simulink model "Induction_motor_Speed_Control_PI"  (R2023a)
settings: Solver=ode23t  StartTime=0.0  StopTime=3  RelTol=1e-3  EnableMultiTasking=on
InitFcn:
  | f=50;
  | fs=2000;
  | %jj=readfis('jayashree1');
libraries: spsAsynchronousMachineSIUnitsLib x1, spsDCVoltageSourceLib x1, simulink x1, powerlib_extras x1, spsThreePhaseVIMeasurementLib x1, spsUniversalBridgeLib x1, sps_lib x1
settings Model: Creator=admin  LastModifiedBy=ravikrishna_g3
settings SolverCC: ZeroCrossControl=DisableAll  AlgebraicLoopSolver=TrustRegion
settings DataIOCC: LimitDataPoints=on  SaveFormat=Array  SignalLoggingSaveFormat=ModelDataLogs  ReturnWorkspaceOutputs=off
settings OptimizationCC: ExpressionDepthLimit=2147483647  LifeSpan=inf
settings DebuggingCC: UnderspecifiedInitializationDetection=Classic  MergeDetectMultiDrivingBlocksExec=none  SolverPrmCheckMsg=warning  FcnCallInpInsideContextMsg=warning  UnconnectedInputMsg=warning  UnconnectedOutputMsg=warning  UnconnectedLineMsg=warning  StateNameClashWarn=warning  SFUnexpectedBacktrackingDiag=warning  SFNoUnconditionalDefaultTransitionDiag=warning  SFExecutionAtInitializationDiag=none  ArithmeticOperatorsInVariantConditions=warning
settings HardwareCC: ProdBitPerPointer=32  ProdBitPerSizeT=32  ProdBitPerPtrDiffT=32  ProdLargestAtomicFloat=None  ProdIntDivRoundTo=Undefined  ProdEndianess=Unspecified  ProdWordSize=32  ProdHWDeviceType=32-bit Generic
settings ModelReferenceCC: PropagateSignalLabelsOutOfModel=off
settings SFSimCC: SimUseLocalCustomCode=off  CustomCodeUndefinedFunction=UseInterfaceOnly
settings RTWCC: RTWUseLocalCustomCode=off
settings CodeAppCC: StateflowObjectComments=on
settings GRTTargetCC: TargetLangStandard=C89/C90 (ANSI)  CombineOutputUpdateFcns=off  GRTInterface=on
settings ConfigComp: CovMetricSettings=dw  CovSaveCumulativeToWorkspaceVar=on  CovSaveSingleToWorkspaceVar=on  CovExternalEMLEnable=off

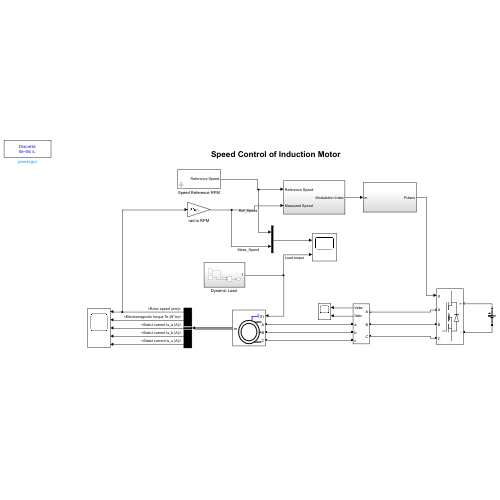
[thumbnail: Simulink's stored preview of the top-level diagram]
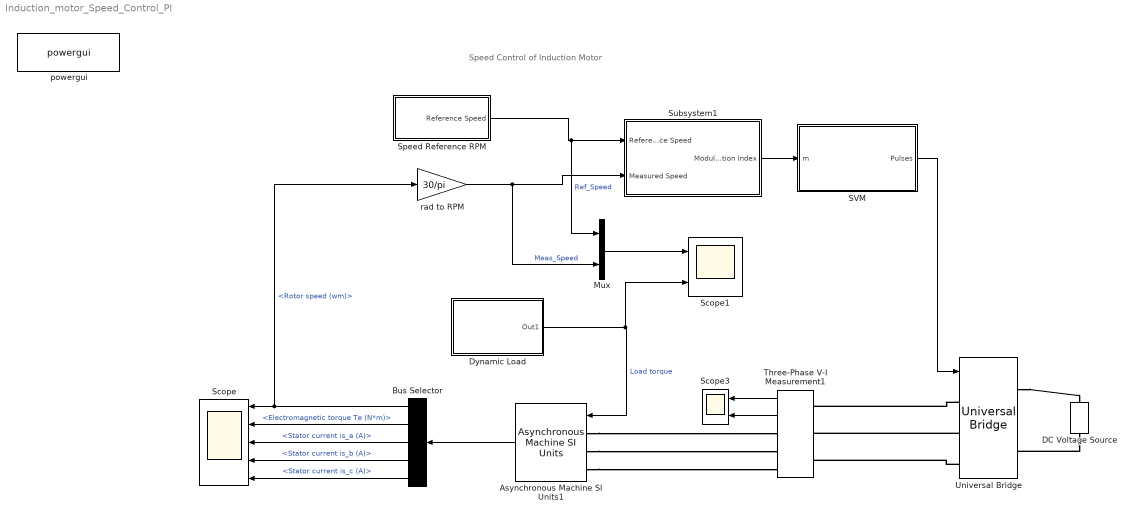
== system Induction_motor_Speed_Control_PI ==
  note: Speed Control of Induction Motor
  Asynchronous Machine SI Units1 : spsAsynchronousMachineSIUnitsLib/Asynchronous Machine SI Units  RotorType=Squirrel-cage  PresetModel="16:  10 HP (7.5KW)  400 V 50Hz 1440 RPM"  MechanicalLoad=Torque Tm  ShowDetailedParameters=on  ReferenceFrame=Rotor  Units=SI  MeasurementBus=off  NominalParameters=[7500 400 50]  VoltageRatio=1  Stator=[0.7384 0.003045]  Rotor=[0.7402 0.003045]  Cage1=[ 0.022 0.226/377]  Cage2=[ 0.022 0.226/377]  Lm=0.1241  Mechanical=[0.0343 0.000503 2]  PolePairs=2  InitialConditions=[1 0 0 0 0 0 0 0]  SimulateSaturation=off  Saturation=[14.03593122, 27.81365428, 53.79336849, 72.68890987, 97.98006896, 148.6815601, 215.7428561, 302.9841135, 428.7778367 ; 230, 322, 414, 460, 506, 552, 598, 644, 690]  LoadFlowParameters=1492000  TsPowergui=0  TsBlock=-1  IterativeModel=Forward Euler  IterativeDiscreteModel=Trapezoidal non iterative  Pmec=0
      settings: AttributesFormatString=\n
  Bus Selector : BusSelector  OutputSignals=Mechanical.Rotor speed (wm),Mechanical.Electromagnetic torque Te (N*m),Stator measurements.Stator current is_a (A),Stator measurements.Stator current is_b (A),Stator measurements.Stator current is_c (A)
  DC Voltage Source : spsDCVoltageSourceLib/DC Voltage Source  Amplitude=400  Measurements=None
  "Dynamic Load " : Subsystem
  Mux : Mux  Inputs=2
  SVM : Subsystem
  Scope : Scope  NumInputPorts=5
  Scope1 : Scope  NumInputPorts=2
  Scope3 : Scope  NumInputPorts=2
  Speed Reference RPM : Subsystem
      mask DialogControl DescTextVar Prompt: Speed
  Subsystem1 : Subsystem
  Three-Phase V-I Measurement1 : spsThreePhaseVIMeasurementLib/Three-Phase V-I Measurement  VoltageMeasurement=phase-to-phase  SetLabelV=off  LabelV=Vabc  Vpu=off  VpuLL=off  CurrentMeasurement=yes  SetLabelI=off  LabelI=Iabc  Ipu=off  Pbase=100e6  Vbase=500e3  OutputType=Complex  PhasorSimulation=off  PSBequivalent=0
  Universal Bridge : spsUniversalBridgeLib/Universal Bridge  Arms=3  SnubberResistance=500  SnubberCapacitance=1e-6  Device=MOSFET / Diodes  Ron=1e-6  Lon=0  ForwardVoltages="[  0  0  ]"  ForwardVoltage=0  GTOparameters=[ 10e-6 , 20e-6 ]  IGBTparameters=[ 1e-6 , 2e-6 ]  Measurements=None  Measurements_2=None  converterType=Rectifier
  powergui : sps_lib/powergui  Priority=1  SimulationMode=Discrete  SampleTime=5e-6  frequency=60  Iterations=50  frequencyindice=50  Pbase=100e6  ErrMax=1e-4  UnitsV=kV  UnitsW=MW  buscounter=0  FunctionMessages=off  echomessages=off  EnableUseOfTLC=off  CurrentSourceSwitches=off  DisableSnubberDevices=off  DisableRonSwitches=off  DisableVfSwitches=off  DisplayEquations=off  AutomaticDiscreteSolvers=off  SolverType=Tustin/Backward Euler (TBE)  Interpol=off  ExternalGateDelay=off  methode=off  Ts=0  x0status=blocks  SPID=off  SwTol=0  HookPort=off  NonlinearTolerance=1e-4  nMaxIteration=100  ContinueOnMaxIteration=off  RestoreLinks=warning  ResistiveCurrentMeasurement=off  Frange=[0:2:500]  Ylog=off  Xlog=on  ShowGrid=off  save=off  variable=ZData  structure=0  ZoomFFT=off  StartTime=0.0  cycles=1  DisplayStyle=1  fundamental=60  FreqAxis=off  MaxFrequency=1000  frequencyindicesteady=1  RmsSteady=1  display=off
  rad to RPM : Gain  Gain=30/pi
  wires:
  Three-Phase V-I Measurement1/2 -> Scope3/2
  Asynchronous Machine SI Units1/1 -> Bus Selector/1
  Three-Phase V-I Measurement1/1 -> Scope3/1
  Bus Selector/1 -> Scope/1, rad to RPM/1  "<Rotor speed (wm)>"
  Bus Selector/2 -> Scope/2  "<Electromagnetic torque Te (N*m)>"
  Bus Selector/3 -> Scope/3  "<Stator current is_a (A)>"
  Bus Selector/4 -> Scope/4  "<Stator current is_b (A)>"
  Bus Selector/5 -> Scope/5  "<Stator current is_c (A)>"
  SVM/1(Pulses) -> Universal Bridge/1
  Subsystem1/1(Modulation Index) -> SVM/1(m)
  "Dynamic Load "/1(Out1) -> Scope1/2, Asynchronous Machine SI Units1/1  "Load torque"
  Speed Reference RPM/1(Reference Speed) -> Mux/1, Subsystem1/1(Reference Speed)  "Ref_Speed"
  rad to RPM/1 -> Subsystem1/2(Measured Speed), Mux/2  "Meas_Speed"
  Mux/1 -> Scope1/1
  connections:
  Universal Bridge/LConn1 -- Three-Phase V-I Measurement1/LConn1
  Universal Bridge/LConn2 -- Three-Phase V-I Measurement1/LConn2
  Universal Bridge/LConn3 -- Three-Phase V-I Measurement1/LConn3
  Asynchronous Machine SI Units1/LConn1 -- Three-Phase V-I Measurement1/RConn1
  Asynchronous Machine SI Units1/LConn3 -- Three-Phase V-I Measurement1/RConn3
  DC Voltage Source/LConn1 -- Universal Bridge/RConn2
  Asynchronous Machine SI Units1/LConn2 -- Three-Phase V-I Measurement1/RConn2
  Universal Bridge/RConn1 -- DC Voltage Source/RConn1

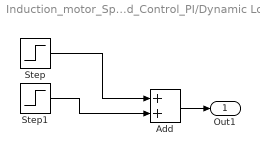
== system Induction_motor_Speed_Control_PI/Dynamic Load  ==
  Add : Sum
  Step : Step  Time=0.2  Before=5  After=10  SampleTime=0
  Step1 : Step  Time=1.2  After=2  SampleTime=0
  Out1 : Outport
  wires:
  Step/1 -> Add/1
  Step1/1 -> Add/2
  Add/1 -> Out1/1

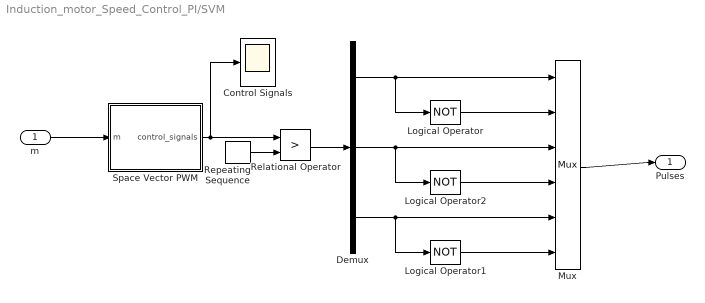
== system Induction_motor_Speed_Control_PI/SVM ==
  m : Inport
  Control Signals : Scope
  Demux : Demux  Outputs=3
  Logical Operator : Logic  Operator=NOT  AllPortsSameDT=off  OutDataTypeStr=boolean
  Logical Operator1 : Logic  Operator=NOT  AllPortsSameDT=off  OutDataTypeStr=boolean
  Logical Operator2 : Logic  Operator=NOT  AllPortsSameDT=off  OutDataTypeStr=boolean
  Mux : Mux  Inputs=6
  Relational Operator : RelationalOperator  Operator=>  InputSameDT=off
  Repeating Sequence : simulink/Sources/Repeating Sequence  rep_seq_t=[0 0.25/fs 0.5/fs 0.75/fs 1/fs]  rep_seq_y=[4 0 -4 0 4]
  Space Vector PWM : Subsystem
  Pulses : Outport
  wires:
  Space Vector PWM/1(control_signals) -> Relational Operator/1, Control Signals/1
  Repeating Sequence/1 -> Relational Operator/2
  Relational Operator/1 -> Demux/1
  Logical Operator/1 -> Mux/2
  Logical Operator2/1 -> Mux/4
  Logical Operator1/1 -> Mux/6
  Demux/1 -> Logical Operator/1, Mux/1
  Demux/2 -> Logical Operator2/1, Mux/3
  Demux/3 -> Logical Operator1/1, Mux/5
  Mux/1 -> Pulses/1
  m/1 -> Space Vector PWM/1(m)

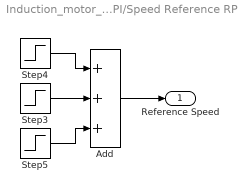
== system Induction_motor_Speed_Control_PI/Speed Reference RPM ==
  Add : Sum  Inputs=+++
  Step3 : Step  Time=1.5  After=50  SampleTime=0
  Step4 : Step  Before=1300  After=1400  SampleTime=0
  Step5 : Step  Time=2  After=-100  SampleTime=0
  Reference Speed : Outport
  wires:
  Add/1 -> Reference Speed/1
  Step5/1 -> Add/3
  Step3/1 -> Add/2
  Step4/1 -> Add/1

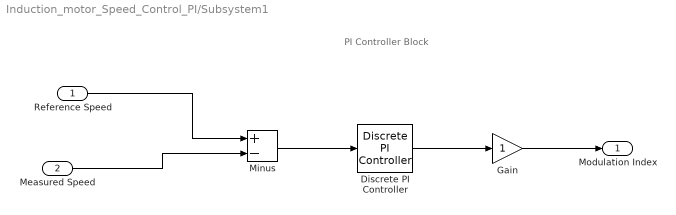
== system Induction_motor_Speed_Control_PI/Subsystem1 ==
  note: PI Controller Block
  Reference Speed : Inport
  Measured Speed : Inport  Port=2
  Discrete PI Controller : powerlib_extras/Discrete  Control Blocks/Discrete PI Controller  Kp=1.2  Ki=0.01  Par_Limits=[4 -4]  Init=0  Ts=50e-6
  Gain : Gain
  Minus : Sum  Inputs=+-
  Modulation Index : Outport
  wires:
  Reference Speed/1 -> Minus/1
  Measured Speed/1 -> Minus/2
  Minus/1 -> Discrete PI Controller/1
  Discrete PI Controller/1 -> Gain/1
  Gain/1 -> Modulation Index/1

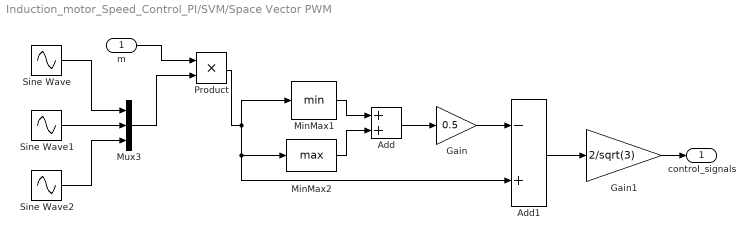
== system Induction_motor_Speed_Control_PI/SVM/Space Vector PWM ==
  m : Inport
  Add : Sum
  Add1 : Sum  Inputs=-+
  Gain : Gain  Gain=0.5
  Gain1 : Gain  Gain=2/sqrt(3)
  MinMax1 : MinMax  InputSameDT=on  SaturateOnIntegerOverflow=on
  MinMax2 : MinMax  Function=max  InputSameDT=on  SaturateOnIntegerOverflow=on
  Mux3 : Mux  Inputs=3
  Product : Product  RndMeth=Zero
  Sine Wave : Sin  Frequency=2*pi*f  Phase=pi/2  SampleTime=0
  Sine Wave1 : Sin  Frequency=2*pi*f  Phase=pi/2 -2*pi/3  SampleTime=0
  Sine Wave2 : Sin  Frequency=2*pi*f  Phase=pi/2+2*pi/3  SampleTime=0
  control_signals : Outport
  wires:
  Sine Wave/1 -> Mux3/1
  Sine Wave1/1 -> Mux3/2
  Sine Wave2/1 -> Mux3/3
  Product/1 -> MinMax1/1, MinMax2/1, Add1/2
  MinMax1/1 -> Add/1
  MinMax2/1 -> Add/2
  Add/1 -> Gain/1
  Gain/1 -> Add1/1
  Add1/1 -> Gain1/1
  Gain1/1 -> control_signals/1
  m/1 -> Product/1
  Mux3/1 -> Product/2
